simulink model "TST_InjSys_Co"  (R2016b)
settings: Solver=FixedStepDiscrete  StartTime=0.0  StopTime=simTime  FixedStep=sampleTime  RelTol=1e-3
values from neighbouring files (symbols this model uses):
  testCase = 1    [initTST_InjSys_Co_001.m]    (also in initTST_InjSys_Co_002.m = 2; initTST_InjSys_Co_003.m = 3; initTST_InjSys_Co_004.m = 4)
libraries: simulink x33, UnitTest_Lib x28
settings Model: Creator=zhengjinyan  LastModifiedBy=zhengjinyan
settings DebuggingCC: SignalRangeChecking=error

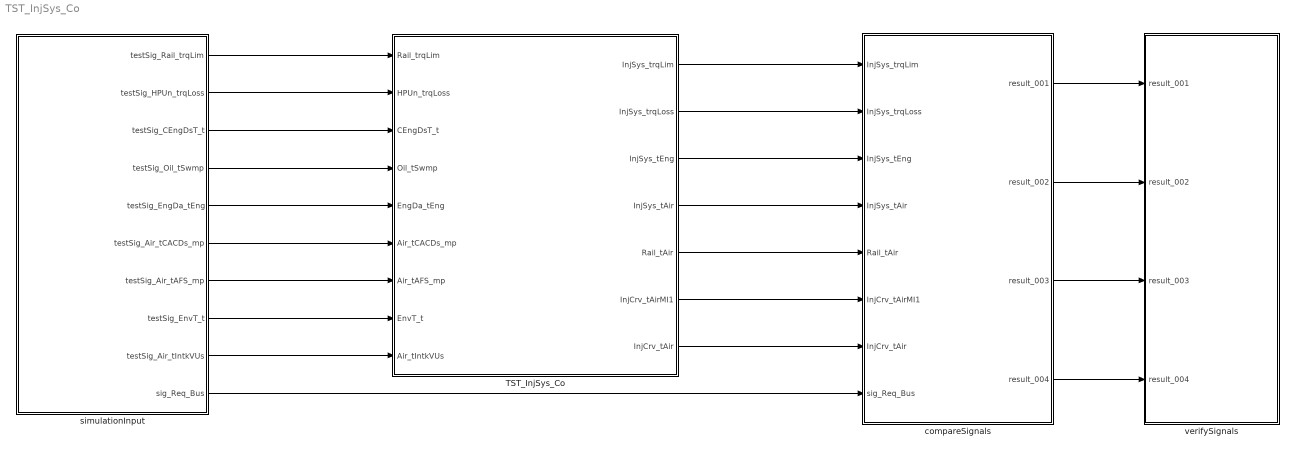
== system TST_InjSys_Co ==
  TST_InjSys_Co : Subsystem
  compareSignals : Subsystem
  simulationInput : Subsystem
  verifySignals : Subsystem
  wires:
  simulationInput/1(testSig_Rail_trqLim) -> TST_InjSys_Co/1(Rail_trqLim)
  simulationInput/2(testSig_HPUn_trqLoss) -> TST_InjSys_Co/2(HPUn_trqLoss)
  simulationInput/3(testSig_CEngDsT_t) -> TST_InjSys_Co/3(CEngDsT_t)
  simulationInput/4(testSig_Oil_tSwmp) -> TST_InjSys_Co/4(Oil_tSwmp)
  simulationInput/5(testSig_EngDa_tEng) -> TST_InjSys_Co/5(EngDa_tEng)
  simulationInput/6(testSig_Air_tCACDs_mp) -> TST_InjSys_Co/6(Air_tCACDs_mp)
  simulationInput/7(testSig_Air_tAFS_mp) -> TST_InjSys_Co/7(Air_tAFS_mp)
  simulationInput/8(testSig_EnvT_t) -> TST_InjSys_Co/8(EnvT_t)
  simulationInput/9(testSig_Air_tIntkVUs) -> TST_InjSys_Co/9(Air_tIntkVUs)
  TST_InjSys_Co/1(InjSys_trqLim) -> compareSignals/1(InjSys_trqLim)
  TST_InjSys_Co/2(InjSys_trqLoss) -> compareSignals/2(InjSys_trqLoss)
  TST_InjSys_Co/3(InjSys_tEng) -> compareSignals/3(InjSys_tEng)
  TST_InjSys_Co/4(InjSys_tAir) -> compareSignals/4(InjSys_tAir)
  TST_InjSys_Co/5(Rail_tAir) -> compareSignals/5(Rail_tAir)
  TST_InjSys_Co/6(InjCrv_tAirMI1) -> compareSignals/6(InjCrv_tAirMI1)
  TST_InjSys_Co/7(InjCrv_tAir) -> compareSignals/7(InjCrv_tAir)
  simulationInput/10(sig_Req_Bus) -> compareSignals/8(sig_Req_Bus)
  compareSignals/1(result_001) -> verifySignals/1(result_001)
  compareSignals/2(result_002) -> verifySignals/2(result_002)
  compareSignals/3(result_003) -> verifySignals/3(result_003)
  compareSignals/4(result_004) -> verifySignals/4(result_004)

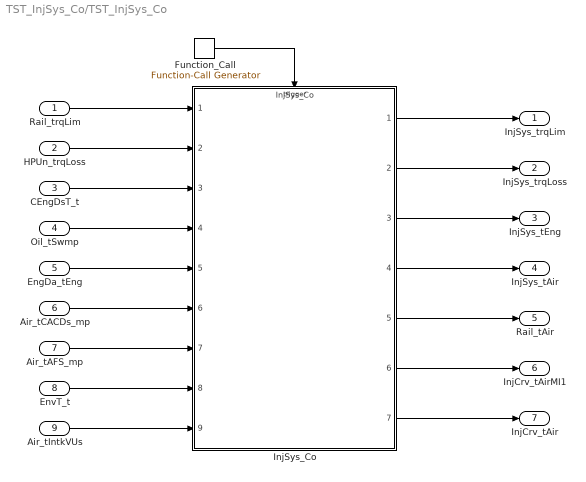
== system TST_InjSys_Co/TST_InjSys_Co ==
  Rail_trqLim : Inport
  HPUn_trqLoss : Inport  Port=2
  CEngDsT_t : Inport  Port=3
  Oil_tSwmp : Inport  Port=4
  EngDa_tEng : Inport  Port=5
  Air_tCACDs_mp : Inport  Port=6
  Air_tAFS_mp : Inport  Port=7
  EnvT_t : Inport  Port=8
  Air_tIntkVUs : Inport  Port=9
  Function_Call : simulink/Ports & Subsystems/Function-Call Generator  sample_time=sampleTime  numberOfIterations=1
  InjSys_Co : ModelReference  ModelNameDialog=InjSys_Co  SimulationMode=Normal  ModelReferenceVersion=1.12  TriggerPortName=function  TriggerPortTriggerType=function-call  TriggerPortStatesWhenEnabling=held
  InjSys_trqLim : Outport
  InjSys_trqLoss : Outport  Port=2
  InjSys_tEng : Outport  Port=3
  InjSys_tAir : Outport  Port=4
  Rail_tAir : Outport  Port=5
  InjCrv_tAirMI1 : Outport  Port=6
  InjCrv_tAir : Outport  Port=7
  wires:
  Function_Call/1 -> InjSys_Co/Trigger
  Rail_trqLim/1 -> InjSys_Co/1
  HPUn_trqLoss/1 -> InjSys_Co/2
  CEngDsT_t/1 -> InjSys_Co/3
  Oil_tSwmp/1 -> InjSys_Co/4
  EngDa_tEng/1 -> InjSys_Co/5
  Air_tCACDs_mp/1 -> InjSys_Co/6
  Air_tAFS_mp/1 -> InjSys_Co/7
  EnvT_t/1 -> InjSys_Co/8
  Air_tIntkVUs/1 -> InjSys_Co/9
  InjSys_Co/1 -> InjSys_trqLim/1
  InjSys_Co/2 -> InjSys_trqLoss/1
  InjSys_Co/3 -> InjSys_tEng/1
  InjSys_Co/4 -> InjSys_tAir/1
  InjSys_Co/5 -> Rail_tAir/1
  InjSys_Co/6 -> InjCrv_tAirMI1/1
  InjSys_Co/7 -> InjCrv_tAir/1

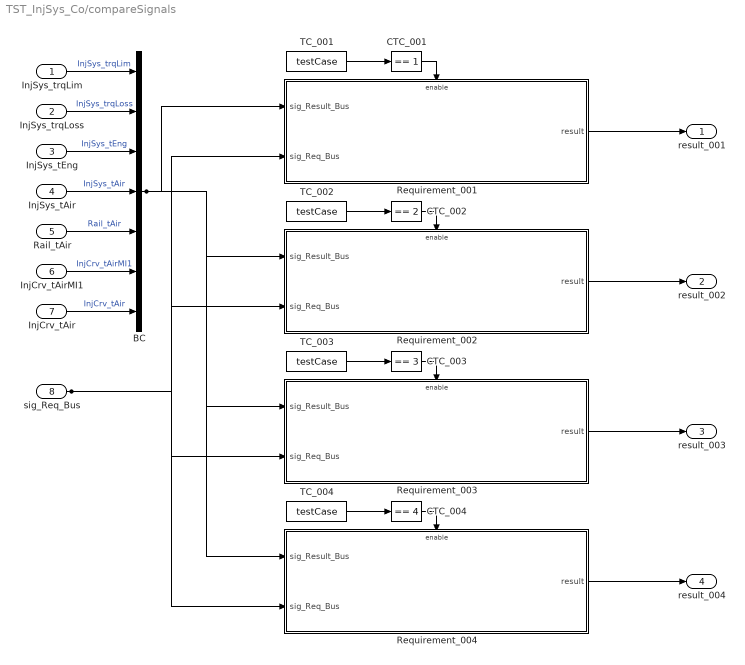
== system TST_InjSys_Co/compareSignals ==
  InjSys_trqLim : Inport
  InjSys_trqLoss : Inport  Port=2
  InjSys_tEng : Inport  Port=3
  InjSys_tAir : Inport  Port=4
  Rail_tAir : Inport  Port=5
  InjCrv_tAirMI1 : Inport  Port=6
  InjCrv_tAir : Inport  Port=7
  sig_Req_Bus : Inport  Port=8
  BC : BusCreator  Inputs=7
  CTC_001 : simulink/Logic and Bit Operations/Compare To Constant  relop===  const=1  OutDataTypeStr=boolean
  CTC_002 : simulink/Logic and Bit Operations/Compare To Constant  relop===  const=2  OutDataTypeStr=boolean
  CTC_003 : simulink/Logic and Bit Operations/Compare To Constant  relop===  const=3  OutDataTypeStr=boolean
  CTC_004 : simulink/Logic and Bit Operations/Compare To Constant  relop===  const=4  OutDataTypeStr=boolean
  Requirement_001 : Subsystem
  Requirement_002 : Subsystem
  Requirement_003 : Subsystem
  Requirement_004 : Subsystem
  TC_001 : Constant  Value=testCase
  TC_002 : Constant  Value=testCase
  TC_003 : Constant  Value=testCase
  TC_004 : Constant  Value=testCase
  result_001 : Outport
  result_002 : Outport  Port=2
  result_003 : Outport  Port=3
  result_004 : Outport  Port=4
  wires:
  InjSys_trqLim/1 -> BC/1  "InjSys_trqLim"
  InjSys_trqLoss/1 -> BC/2  "InjSys_trqLoss"
  InjSys_tEng/1 -> BC/3  "InjSys_tEng"
  InjSys_tAir/1 -> BC/4  "InjSys_tAir"
  Rail_tAir/1 -> BC/5  "Rail_tAir"
  InjCrv_tAirMI1/1 -> BC/6  "InjCrv_tAirMI1"
  InjCrv_tAir/1 -> BC/7  "InjCrv_tAir"
  TC_001/1 -> CTC_001/1
  CTC_001/1 -> Requirement_001/Enable
  sig_Req_Bus/1 -> Requirement_001/2(sig_Req_Bus), Requirement_002/2(sig_Req_Bus), Requirement_003/2(sig_Req_Bus), Requirement_004/2(sig_Req_Bus)
  BC/1 -> Requirement_001/1(sig_Result_Bus), Requirement_002/1(sig_Result_Bus), Requirement_003/1(sig_Result_Bus), Requirement_004/1(sig_Result_Bus)
  Requirement_001/1(result) -> result_001/1
  TC_002/1 -> CTC_002/1
  CTC_002/1 -> Requirement_002/Enable
  Requirement_002/1(result) -> result_002/1
  TC_003/1 -> CTC_003/1
  CTC_003/1 -> Requirement_003/Enable
  Requirement_003/1(result) -> result_003/1
  TC_004/1 -> CTC_004/1
  CTC_004/1 -> Requirement_004/Enable
  Requirement_004/1(result) -> result_004/1

== system TST_InjSys_Co/simulationInput ==
  BS : BusSelector  OutputSignals=testSig_Rail_trqLim,testSig_HPUn_trqLoss,testSig_CEngDsT_t,testSig_Oil_tSwmp,testSig_EngDa_tEng,testSig_Air_tCACDs_mp,testSig_Air_tAFS_mp,testSig_EnvT_t,testSig_Air_tIntkVUs
  MPSw : MultiPortSwitch  Inputs=4  SaturateOnIntegerOverflow=on  InputSameDT=on
  TestCase : Constant  Value=testCase
  testSignals_R001 : Subsystem
  testSignals_R002 : Subsystem
  testSignals_R003 : Subsystem
  testSignals_R004 : Subsystem
  testSig_Rail_trqLim : Outport
  testSig_HPUn_trqLoss : Outport  Port=2
  testSig_CEngDsT_t : Outport  Port=3
  testSig_Oil_tSwmp : Outport  Port=4
  testSig_EngDa_tEng : Outport  Port=5
  testSig_Air_tCACDs_mp : Outport  Port=6
  testSig_Air_tAFS_mp : Outport  Port=7
  testSig_EnvT_t : Outport  Port=8
  testSig_Air_tIntkVUs : Outport  Port=9
  sig_Req_Bus : Outport  Port=10
  wires:
  BS/1 -> testSig_Rail_trqLim/1  "<testSig_Rail_trqLim>"
  BS/2 -> testSig_HPUn_trqLoss/1  "<testSig_HPUn_trqLoss>"
  BS/3 -> testSig_CEngDsT_t/1  "<testSig_CEngDsT_t>"
  BS/4 -> testSig_Oil_tSwmp/1  "<testSig_Oil_tSwmp>"
  BS/5 -> testSig_EngDa_tEng/1  "<testSig_EngDa_tEng>"
  BS/6 -> testSig_Air_tCACDs_mp/1  "<testSig_Air_tCACDs_mp>"
  BS/7 -> testSig_Air_tAFS_mp/1  "<testSig_Air_tAFS_mp>"
  BS/8 -> testSig_EnvT_t/1  "<testSig_EnvT_t>"
  BS/9 -> testSig_Air_tIntkVUs/1  "<testSig_Air_tIntkVUs>"
  MPSw/1 -> BS/1, sig_Req_Bus/1
  TestCase/1 -> MPSw/1
  testSignals_R001/1(testSignals) -> MPSw/2
  testSignals_R002/1(testSignals) -> MPSw/3
  testSignals_R003/1(testSignals) -> MPSw/4
  testSignals_R004/1(testSignals) -> MPSw/5

== system TST_InjSys_Co/verifySignals ==
  result_001 : Inport
  result_002 : Inport  Port=2
  result_003 : Inport  Port=3
  result_004 : Inport  Port=4
  Assertion_001 : Assertion  Enabled=off
  Assertion_002 : Assertion  Enabled=off
  Assertion_003 : Assertion  Enabled=off
  Assertion_004 : Assertion  Enabled=off
  wires:
  result_001/1 -> Assertion_001/1
  result_002/1 -> Assertion_002/1
  result_003/1 -> Assertion_003/1
  result_004/1 -> Assertion_004/1

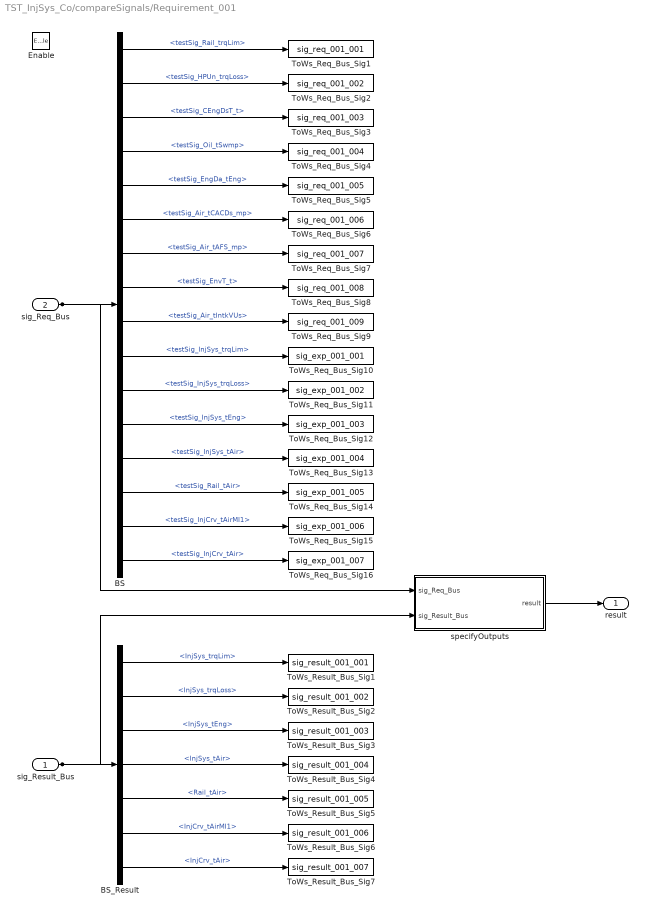
== system TST_InjSys_Co/compareSignals/Requirement_001 ==
  sig_Result_Bus : Inport
  sig_Req_Bus : Inport  Port=2
  Enable : EnablePort
  BS : BusSelector  OutputSignals=testSig_Rail_trqLim,testSig_HPUn_trqLoss,testSig_CEngDsT_t,testSig_Oil_tSwmp,testSig_EngDa_tEng,testSig_Air_tCACDs_mp,testSig_Air_tAFS_mp,testSig_EnvT_t,testSig_Air_tIntkVUs,testSig_InjSys_trqLim,testSig_InjSys_trqLoss,testSig_InjSys_tEng,testSig_InjSys_tAir,testSig_Rail_tAir,testSig_InjCrv_tAirMI1,testSig_InjCrv_tAir
  BS_Result : BusSelector  OutputSignals=InjSys_trqLim,InjSys_trqLoss,InjSys_tEng,InjSys_tAir,Rail_tAir,InjCrv_tAirMI1,InjCrv_tAir
  ToWs_Req_Bus_Sig1 : ToWorkspace  VariableName=sig_req_001_001  SaveFormat=Structure With Time
  ToWs_Req_Bus_Sig10 : ToWorkspace  VariableName=sig_exp_001_001  SaveFormat=Structure With Time
  ToWs_Req_Bus_Sig11 : ToWorkspace  VariableName=sig_exp_001_002  SaveFormat=Structure With Time
  ToWs_Req_Bus_Sig12 : ToWorkspace  VariableName=sig_exp_001_003  SaveFormat=Structure With Time
  ToWs_Req_Bus_Sig13 : ToWorkspace  VariableName=sig_exp_001_004  SaveFormat=Structure With Time
  ToWs_Req_Bus_Sig14 : ToWorkspace  VariableName=sig_exp_001_005  SaveFormat=Structure With Time
  ToWs_Req_Bus_Sig15 : ToWorkspace  VariableName=sig_exp_001_006  SaveFormat=Structure With Time
  ToWs_Req_Bus_Sig16 : ToWorkspace  VariableName=sig_exp_001_007  SaveFormat=Structure With Time
  ToWs_Req_Bus_Sig2 : ToWorkspace  VariableName=sig_req_001_002  SaveFormat=Structure With Time
  ToWs_Req_Bus_Sig3 : ToWorkspace  VariableName=sig_req_001_003  SaveFormat=Structure With Time
  ToWs_Req_Bus_Sig4 : ToWorkspace  VariableName=sig_req_001_004  SaveFormat=Structure With Time
  ToWs_Req_Bus_Sig5 : ToWorkspace  VariableName=sig_req_001_005  SaveFormat=Structure With Time
  ToWs_Req_Bus_Sig6 : ToWorkspace  VariableName=sig_req_001_006  SaveFormat=Structure With Time
  ToWs_Req_Bus_Sig7 : ToWorkspace  VariableName=sig_req_001_007  SaveFormat=Structure With Time
  ToWs_Req_Bus_Sig8 : ToWorkspace  VariableName=sig_req_001_008  SaveFormat=Structure With Time
  ToWs_Req_Bus_Sig9 : ToWorkspace  VariableName=sig_req_001_009  SaveFormat=Structure With Time
  ToWs_Result_Bus_Sig1 : ToWorkspace  VariableName=sig_result_001_001  SaveFormat=Structure With Time
  ToWs_Result_Bus_Sig2 : ToWorkspace  VariableName=sig_result_001_002  SaveFormat=Structure With Time
  ToWs_Result_Bus_Sig3 : ToWorkspace  VariableName=sig_result_001_003  SaveFormat=Structure With Time
  ToWs_Result_Bus_Sig4 : ToWorkspace  VariableName=sig_result_001_004  SaveFormat=Structure With Time
  ToWs_Result_Bus_Sig5 : ToWorkspace  VariableName=sig_result_001_005  SaveFormat=Structure With Time
  ToWs_Result_Bus_Sig6 : ToWorkspace  VariableName=sig_result_001_006  SaveFormat=Structure With Time
  ToWs_Result_Bus_Sig7 : ToWorkspace  VariableName=sig_result_001_007  SaveFormat=Structure With Time
  specifyOutputs : Subsystem
  result : Outport
  wires:
  sig_Req_Bus/1 -> BS/1, specifyOutputs/1(sig_Req_Bus)
  BS/1 -> ToWs_Req_Bus_Sig1/1  "<testSig_Rail_trqLim>"
  BS/2 -> ToWs_Req_Bus_Sig2/1  "<testSig_HPUn_trqLoss>"
  BS/3 -> ToWs_Req_Bus_Sig3/1  "<testSig_CEngDsT_t>"
  BS/4 -> ToWs_Req_Bus_Sig4/1  "<testSig_Oil_tSwmp>"
  BS/5 -> ToWs_Req_Bus_Sig5/1  "<testSig_EngDa_tEng>"
  BS/6 -> ToWs_Req_Bus_Sig6/1  "<testSig_Air_tCACDs_mp>"
  BS/7 -> ToWs_Req_Bus_Sig7/1  "<testSig_Air_tAFS_mp>"
  BS/8 -> ToWs_Req_Bus_Sig8/1  "<testSig_EnvT_t>"
  BS/9 -> ToWs_Req_Bus_Sig9/1  "<testSig_Air_tIntkVUs>"
  BS/10 -> ToWs_Req_Bus_Sig10/1  "<testSig_InjSys_trqLim>"
  BS/11 -> ToWs_Req_Bus_Sig11/1  "<testSig_InjSys_trqLoss>"
  BS/12 -> ToWs_Req_Bus_Sig12/1  "<testSig_InjSys_tEng>"
  BS/13 -> ToWs_Req_Bus_Sig13/1  "<testSig_InjSys_tAir>"
  BS/14 -> ToWs_Req_Bus_Sig14/1  "<testSig_Rail_tAir>"
  BS/15 -> ToWs_Req_Bus_Sig15/1  "<testSig_InjCrv_tAirMI1>"
  BS/16 -> ToWs_Req_Bus_Sig16/1  "<testSig_InjCrv_tAir>"
  sig_Result_Bus/1 -> BS_Result/1, specifyOutputs/2(sig_Result_Bus)
  BS_Result/1 -> ToWs_Result_Bus_Sig1/1  "<InjSys_trqLim>"
  BS_Result/2 -> ToWs_Result_Bus_Sig2/1  "<InjSys_trqLoss>"
  BS_Result/3 -> ToWs_Result_Bus_Sig3/1  "<InjSys_tEng>"
  BS_Result/4 -> ToWs_Result_Bus_Sig4/1  "<InjSys_tAir>"
  BS_Result/5 -> ToWs_Result_Bus_Sig5/1  "<Rail_tAir>"
  BS_Result/6 -> ToWs_Result_Bus_Sig6/1  "<InjCrv_tAirMI1>"
  BS_Result/7 -> ToWs_Result_Bus_Sig7/1  "<InjCrv_tAir>"
  specifyOutputs/1(result) -> result/1

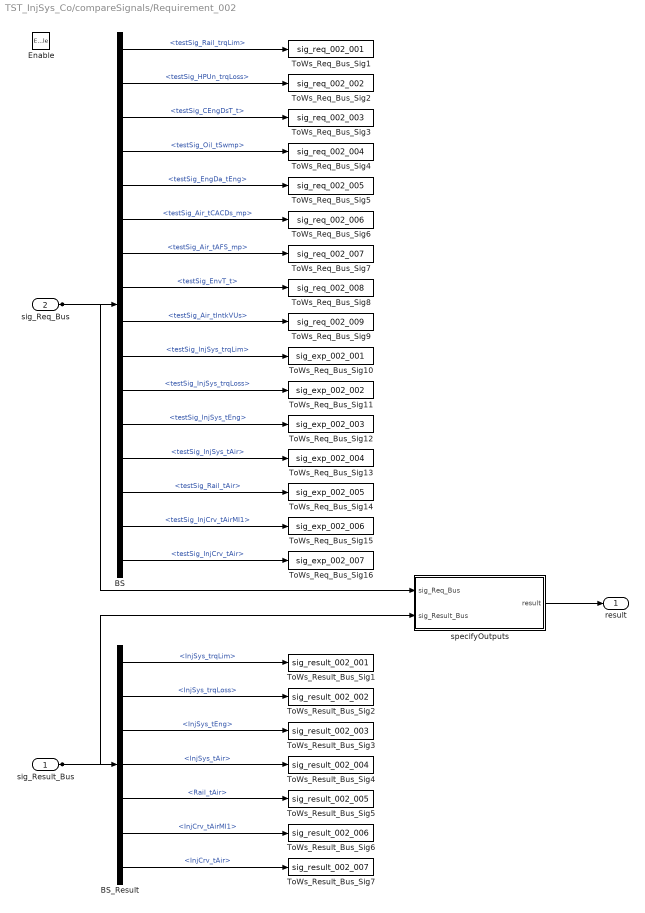
== system TST_InjSys_Co/compareSignals/Requirement_002 ==
  sig_Result_Bus : Inport
  sig_Req_Bus : Inport  Port=2
  Enable : EnablePort
  BS : BusSelector  OutputSignals=testSig_Rail_trqLim,testSig_HPUn_trqLoss,testSig_CEngDsT_t,testSig_Oil_tSwmp,testSig_EngDa_tEng,testSig_Air_tCACDs_mp,testSig_Air_tAFS_mp,testSig_EnvT_t,testSig_Air_tIntkVUs,testSig_InjSys_trqLim,testSig_InjSys_trqLoss,testSig_InjSys_tEng,testSig_InjSys_tAir,testSig_Rail_tAir,testSig_InjCrv_tAirMI1,testSig_InjCrv_tAir
  BS_Result : BusSelector  OutputSignals=InjSys_trqLim,InjSys_trqLoss,InjSys_tEng,InjSys_tAir,Rail_tAir,InjCrv_tAirMI1,InjCrv_tAir
  ToWs_Req_Bus_Sig1 : ToWorkspace  VariableName=sig_req_002_001  SaveFormat=Structure With Time
  ToWs_Req_Bus_Sig10 : ToWorkspace  VariableName=sig_exp_002_001  SaveFormat=Structure With Time
  ToWs_Req_Bus_Sig11 : ToWorkspace  VariableName=sig_exp_002_002  SaveFormat=Structure With Time
  ToWs_Req_Bus_Sig12 : ToWorkspace  VariableName=sig_exp_002_003  SaveFormat=Structure With Time
  ToWs_Req_Bus_Sig13 : ToWorkspace  VariableName=sig_exp_002_004  SaveFormat=Structure With Time
  ToWs_Req_Bus_Sig14 : ToWorkspace  VariableName=sig_exp_002_005  SaveFormat=Structure With Time
  ToWs_Req_Bus_Sig15 : ToWorkspace  VariableName=sig_exp_002_006  SaveFormat=Structure With Time
  ToWs_Req_Bus_Sig16 : ToWorkspace  VariableName=sig_exp_002_007  SaveFormat=Structure With Time
  ToWs_Req_Bus_Sig2 : ToWorkspace  VariableName=sig_req_002_002  SaveFormat=Structure With Time
  ToWs_Req_Bus_Sig3 : ToWorkspace  VariableName=sig_req_002_003  SaveFormat=Structure With Time
  ToWs_Req_Bus_Sig4 : ToWorkspace  VariableName=sig_req_002_004  SaveFormat=Structure With Time
  ToWs_Req_Bus_Sig5 : ToWorkspace  VariableName=sig_req_002_005  SaveFormat=Structure With Time
  ToWs_Req_Bus_Sig6 : ToWorkspace  VariableName=sig_req_002_006  SaveFormat=Structure With Time
  ToWs_Req_Bus_Sig7 : ToWorkspace  VariableName=sig_req_002_007  SaveFormat=Structure With Time
  ToWs_Req_Bus_Sig8 : ToWorkspace  VariableName=sig_req_002_008  SaveFormat=Structure With Time
  ToWs_Req_Bus_Sig9 : ToWorkspace  VariableName=sig_req_002_009  SaveFormat=Structure With Time
  ToWs_Result_Bus_Sig1 : ToWorkspace  VariableName=sig_result_002_001  SaveFormat=Structure With Time
  ToWs_Result_Bus_Sig2 : ToWorkspace  VariableName=sig_result_002_002  SaveFormat=Structure With Time
  ToWs_Result_Bus_Sig3 : ToWorkspace  VariableName=sig_result_002_003  SaveFormat=Structure With Time
  ToWs_Result_Bus_Sig4 : ToWorkspace  VariableName=sig_result_002_004  SaveFormat=Structure With Time
  ToWs_Result_Bus_Sig5 : ToWorkspace  VariableName=sig_result_002_005  SaveFormat=Structure With Time
  ToWs_Result_Bus_Sig6 : ToWorkspace  VariableName=sig_result_002_006  SaveFormat=Structure With Time
  ToWs_Result_Bus_Sig7 : ToWorkspace  VariableName=sig_result_002_007  SaveFormat=Structure With Time
  specifyOutputs : Subsystem
  result : Outport
  wires:
  sig_Req_Bus/1 -> BS/1, specifyOutputs/1(sig_Req_Bus)
  BS/1 -> ToWs_Req_Bus_Sig1/1  "<testSig_Rail_trqLim>"
  BS/2 -> ToWs_Req_Bus_Sig2/1  "<testSig_HPUn_trqLoss>"
  BS/3 -> ToWs_Req_Bus_Sig3/1  "<testSig_CEngDsT_t>"
  BS/4 -> ToWs_Req_Bus_Sig4/1  "<testSig_Oil_tSwmp>"
  BS/5 -> ToWs_Req_Bus_Sig5/1  "<testSig_EngDa_tEng>"
  BS/6 -> ToWs_Req_Bus_Sig6/1  "<testSig_Air_tCACDs_mp>"
  BS/7 -> ToWs_Req_Bus_Sig7/1  "<testSig_Air_tAFS_mp>"
  BS/8 -> ToWs_Req_Bus_Sig8/1  "<testSig_EnvT_t>"
  BS/9 -> ToWs_Req_Bus_Sig9/1  "<testSig_Air_tIntkVUs>"
  BS/10 -> ToWs_Req_Bus_Sig10/1  "<testSig_InjSys_trqLim>"
  BS/11 -> ToWs_Req_Bus_Sig11/1  "<testSig_InjSys_trqLoss>"
  BS/12 -> ToWs_Req_Bus_Sig12/1  "<testSig_InjSys_tEng>"
  BS/13 -> ToWs_Req_Bus_Sig13/1  "<testSig_InjSys_tAir>"
  BS/14 -> ToWs_Req_Bus_Sig14/1  "<testSig_Rail_tAir>"
  BS/15 -> ToWs_Req_Bus_Sig15/1  "<testSig_InjCrv_tAirMI1>"
  BS/16 -> ToWs_Req_Bus_Sig16/1  "<testSig_InjCrv_tAir>"
  sig_Result_Bus/1 -> BS_Result/1, specifyOutputs/2(sig_Result_Bus)
  BS_Result/1 -> ToWs_Result_Bus_Sig1/1  "<InjSys_trqLim>"
  BS_Result/2 -> ToWs_Result_Bus_Sig2/1  "<InjSys_trqLoss>"
  BS_Result/3 -> ToWs_Result_Bus_Sig3/1  "<InjSys_tEng>"
  BS_Result/4 -> ToWs_Result_Bus_Sig4/1  "<InjSys_tAir>"
  BS_Result/5 -> ToWs_Result_Bus_Sig5/1  "<Rail_tAir>"
  BS_Result/6 -> ToWs_Result_Bus_Sig6/1  "<InjCrv_tAirMI1>"
  BS_Result/7 -> ToWs_Result_Bus_Sig7/1  "<InjCrv_tAir>"
  specifyOutputs/1(result) -> result/1

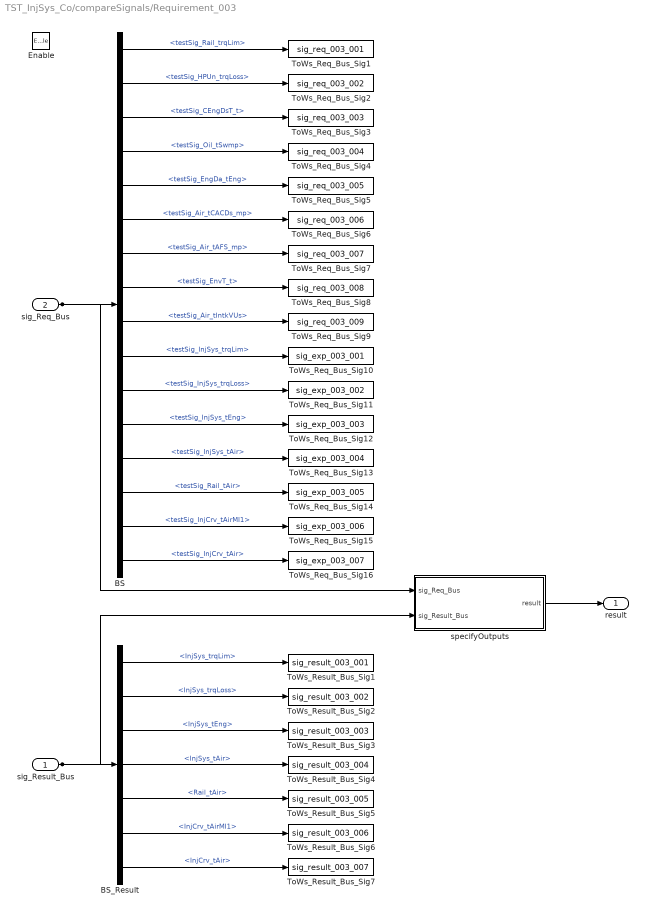
== system TST_InjSys_Co/compareSignals/Requirement_003 ==
  sig_Result_Bus : Inport
  sig_Req_Bus : Inport  Port=2
  Enable : EnablePort
  BS : BusSelector  OutputSignals=testSig_Rail_trqLim,testSig_HPUn_trqLoss,testSig_CEngDsT_t,testSig_Oil_tSwmp,testSig_EngDa_tEng,testSig_Air_tCACDs_mp,testSig_Air_tAFS_mp,testSig_EnvT_t,testSig_Air_tIntkVUs,testSig_InjSys_trqLim,testSig_InjSys_trqLoss,testSig_InjSys_tEng,testSig_InjSys_tAir,testSig_Rail_tAir,testSig_InjCrv_tAirMI1,testSig_InjCrv_tAir
  BS_Result : BusSelector  OutputSignals=InjSys_trqLim,InjSys_trqLoss,InjSys_tEng,InjSys_tAir,Rail_tAir,InjCrv_tAirMI1,InjCrv_tAir
  ToWs_Req_Bus_Sig1 : ToWorkspace  VariableName=sig_req_003_001  SaveFormat=Structure With Time
  ToWs_Req_Bus_Sig10 : ToWorkspace  VariableName=sig_exp_003_001  SaveFormat=Structure With Time
  ToWs_Req_Bus_Sig11 : ToWorkspace  VariableName=sig_exp_003_002  SaveFormat=Structure With Time
  ToWs_Req_Bus_Sig12 : ToWorkspace  VariableName=sig_exp_003_003  SaveFormat=Structure With Time
  ToWs_Req_Bus_Sig13 : ToWorkspace  VariableName=sig_exp_003_004  SaveFormat=Structure With Time
  ToWs_Req_Bus_Sig14 : ToWorkspace  VariableName=sig_exp_003_005  SaveFormat=Structure With Time
  ToWs_Req_Bus_Sig15 : ToWorkspace  VariableName=sig_exp_003_006  SaveFormat=Structure With Time
  ToWs_Req_Bus_Sig16 : ToWorkspace  VariableName=sig_exp_003_007  SaveFormat=Structure With Time
  ToWs_Req_Bus_Sig2 : ToWorkspace  VariableName=sig_req_003_002  SaveFormat=Structure With Time
  ToWs_Req_Bus_Sig3 : ToWorkspace  VariableName=sig_req_003_003  SaveFormat=Structure With Time
  ToWs_Req_Bus_Sig4 : ToWorkspace  VariableName=sig_req_003_004  SaveFormat=Structure With Time
  ToWs_Req_Bus_Sig5 : ToWorkspace  VariableName=sig_req_003_005  SaveFormat=Structure With Time
  ToWs_Req_Bus_Sig6 : ToWorkspace  VariableName=sig_req_003_006  SaveFormat=Structure With Time
  ToWs_Req_Bus_Sig7 : ToWorkspace  VariableName=sig_req_003_007  SaveFormat=Structure With Time
  ToWs_Req_Bus_Sig8 : ToWorkspace  VariableName=sig_req_003_008  SaveFormat=Structure With Time
  ToWs_Req_Bus_Sig9 : ToWorkspace  VariableName=sig_req_003_009  SaveFormat=Structure With Time
  ToWs_Result_Bus_Sig1 : ToWorkspace  VariableName=sig_result_003_001  SaveFormat=Structure With Time
  ToWs_Result_Bus_Sig2 : ToWorkspace  VariableName=sig_result_003_002  SaveFormat=Structure With Time
  ToWs_Result_Bus_Sig3 : ToWorkspace  VariableName=sig_result_003_003  SaveFormat=Structure With Time
  ToWs_Result_Bus_Sig4 : ToWorkspace  VariableName=sig_result_003_004  SaveFormat=Structure With Time
  ToWs_Result_Bus_Sig5 : ToWorkspace  VariableName=sig_result_003_005  SaveFormat=Structure With Time
  ToWs_Result_Bus_Sig6 : ToWorkspace  VariableName=sig_result_003_006  SaveFormat=Structure With Time
  ToWs_Result_Bus_Sig7 : ToWorkspace  VariableName=sig_result_003_007  SaveFormat=Structure With Time
  specifyOutputs : Subsystem
  result : Outport
  wires:
  sig_Req_Bus/1 -> BS/1, specifyOutputs/1(sig_Req_Bus)
  BS/1 -> ToWs_Req_Bus_Sig1/1  "<testSig_Rail_trqLim>"
  BS/2 -> ToWs_Req_Bus_Sig2/1  "<testSig_HPUn_trqLoss>"
  BS/3 -> ToWs_Req_Bus_Sig3/1  "<testSig_CEngDsT_t>"
  BS/4 -> ToWs_Req_Bus_Sig4/1  "<testSig_Oil_tSwmp>"
  BS/5 -> ToWs_Req_Bus_Sig5/1  "<testSig_EngDa_tEng>"
  BS/6 -> ToWs_Req_Bus_Sig6/1  "<testSig_Air_tCACDs_mp>"
  BS/7 -> ToWs_Req_Bus_Sig7/1  "<testSig_Air_tAFS_mp>"
  BS/8 -> ToWs_Req_Bus_Sig8/1  "<testSig_EnvT_t>"
  BS/9 -> ToWs_Req_Bus_Sig9/1  "<testSig_Air_tIntkVUs>"
  BS/10 -> ToWs_Req_Bus_Sig10/1  "<testSig_InjSys_trqLim>"
  BS/11 -> ToWs_Req_Bus_Sig11/1  "<testSig_InjSys_trqLoss>"
  BS/12 -> ToWs_Req_Bus_Sig12/1  "<testSig_InjSys_tEng>"
  BS/13 -> ToWs_Req_Bus_Sig13/1  "<testSig_InjSys_tAir>"
  BS/14 -> ToWs_Req_Bus_Sig14/1  "<testSig_Rail_tAir>"
  BS/15 -> ToWs_Req_Bus_Sig15/1  "<testSig_InjCrv_tAirMI1>"
  BS/16 -> ToWs_Req_Bus_Sig16/1  "<testSig_InjCrv_tAir>"
  sig_Result_Bus/1 -> BS_Result/1, specifyOutputs/2(sig_Result_Bus)
  BS_Result/1 -> ToWs_Result_Bus_Sig1/1  "<InjSys_trqLim>"
  BS_Result/2 -> ToWs_Result_Bus_Sig2/1  "<InjSys_trqLoss>"
  BS_Result/3 -> ToWs_Result_Bus_Sig3/1  "<InjSys_tEng>"
  BS_Result/4 -> ToWs_Result_Bus_Sig4/1  "<InjSys_tAir>"
  BS_Result/5 -> ToWs_Result_Bus_Sig5/1  "<Rail_tAir>"
  BS_Result/6 -> ToWs_Result_Bus_Sig6/1  "<InjCrv_tAirMI1>"
  BS_Result/7 -> ToWs_Result_Bus_Sig7/1  "<InjCrv_tAir>"
  specifyOutputs/1(result) -> result/1

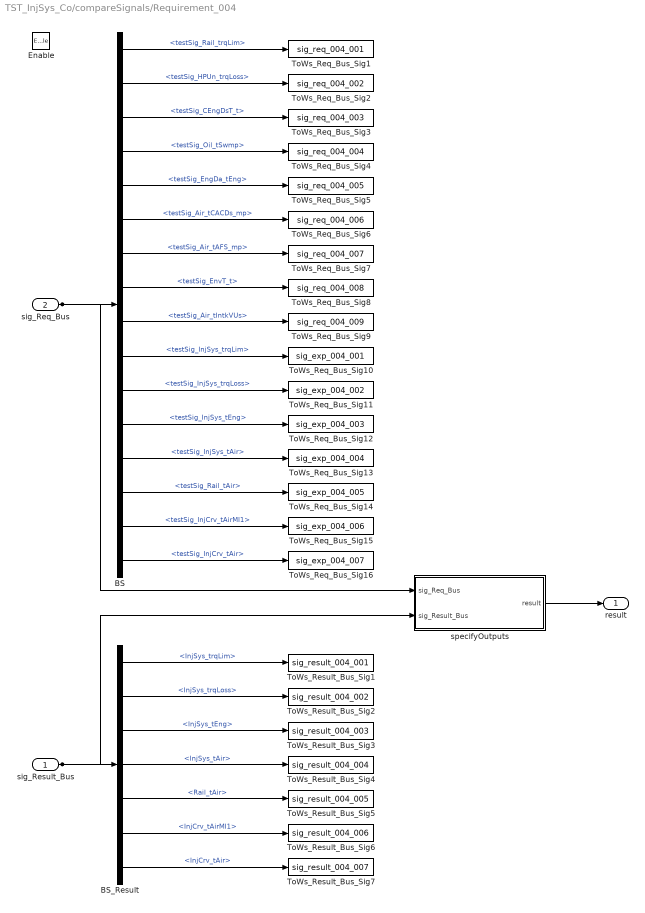
== system TST_InjSys_Co/compareSignals/Requirement_004 ==
  sig_Result_Bus : Inport
  sig_Req_Bus : Inport  Port=2
  Enable : EnablePort
  BS : BusSelector  OutputSignals=testSig_Rail_trqLim,testSig_HPUn_trqLoss,testSig_CEngDsT_t,testSig_Oil_tSwmp,testSig_EngDa_tEng,testSig_Air_tCACDs_mp,testSig_Air_tAFS_mp,testSig_EnvT_t,testSig_Air_tIntkVUs,testSig_InjSys_trqLim,testSig_InjSys_trqLoss,testSig_InjSys_tEng,testSig_InjSys_tAir,testSig_Rail_tAir,testSig_InjCrv_tAirMI1,testSig_InjCrv_tAir
  BS_Result : BusSelector  OutputSignals=InjSys_trqLim,InjSys_trqLoss,InjSys_tEng,InjSys_tAir,Rail_tAir,InjCrv_tAirMI1,InjCrv_tAir
  ToWs_Req_Bus_Sig1 : ToWorkspace  VariableName=sig_req_004_001  SaveFormat=Structure With Time
  ToWs_Req_Bus_Sig10 : ToWorkspace  VariableName=sig_exp_004_001  SaveFormat=Structure With Time
  ToWs_Req_Bus_Sig11 : ToWorkspace  VariableName=sig_exp_004_002  SaveFormat=Structure With Time
  ToWs_Req_Bus_Sig12 : ToWorkspace  VariableName=sig_exp_004_003  SaveFormat=Structure With Time
  ToWs_Req_Bus_Sig13 : ToWorkspace  VariableName=sig_exp_004_004  SaveFormat=Structure With Time
  ToWs_Req_Bus_Sig14 : ToWorkspace  VariableName=sig_exp_004_005  SaveFormat=Structure With Time
  ToWs_Req_Bus_Sig15 : ToWorkspace  VariableName=sig_exp_004_006  SaveFormat=Structure With Time
  ToWs_Req_Bus_Sig16 : ToWorkspace  VariableName=sig_exp_004_007  SaveFormat=Structure With Time
  ToWs_Req_Bus_Sig2 : ToWorkspace  VariableName=sig_req_004_002  SaveFormat=Structure With Time
  ToWs_Req_Bus_Sig3 : ToWorkspace  VariableName=sig_req_004_003  SaveFormat=Structure With Time
  ToWs_Req_Bus_Sig4 : ToWorkspace  VariableName=sig_req_004_004  SaveFormat=Structure With Time
  ToWs_Req_Bus_Sig5 : ToWorkspace  VariableName=sig_req_004_005  SaveFormat=Structure With Time
  ToWs_Req_Bus_Sig6 : ToWorkspace  VariableName=sig_req_004_006  SaveFormat=Structure With Time
  ToWs_Req_Bus_Sig7 : ToWorkspace  VariableName=sig_req_004_007  SaveFormat=Structure With Time
  ToWs_Req_Bus_Sig8 : ToWorkspace  VariableName=sig_req_004_008  SaveFormat=Structure With Time
  ToWs_Req_Bus_Sig9 : ToWorkspace  VariableName=sig_req_004_009  SaveFormat=Structure With Time
  ToWs_Result_Bus_Sig1 : ToWorkspace  VariableName=sig_result_004_001  SaveFormat=Structure With Time
  ToWs_Result_Bus_Sig2 : ToWorkspace  VariableName=sig_result_004_002  SaveFormat=Structure With Time
  ToWs_Result_Bus_Sig3 : ToWorkspace  VariableName=sig_result_004_003  SaveFormat=Structure With Time
  ToWs_Result_Bus_Sig4 : ToWorkspace  VariableName=sig_result_004_004  SaveFormat=Structure With Time
  ToWs_Result_Bus_Sig5 : ToWorkspace  VariableName=sig_result_004_005  SaveFormat=Structure With Time
  ToWs_Result_Bus_Sig6 : ToWorkspace  VariableName=sig_result_004_006  SaveFormat=Structure With Time
  ToWs_Result_Bus_Sig7 : ToWorkspace  VariableName=sig_result_004_007  SaveFormat=Structure With Time
  specifyOutputs : Subsystem
  result : Outport
  wires:
  sig_Req_Bus/1 -> BS/1, specifyOutputs/1(sig_Req_Bus)
  BS/1 -> ToWs_Req_Bus_Sig1/1  "<testSig_Rail_trqLim>"
  BS/2 -> ToWs_Req_Bus_Sig2/1  "<testSig_HPUn_trqLoss>"
  BS/3 -> ToWs_Req_Bus_Sig3/1  "<testSig_CEngDsT_t>"
  BS/4 -> ToWs_Req_Bus_Sig4/1  "<testSig_Oil_tSwmp>"
  BS/5 -> ToWs_Req_Bus_Sig5/1  "<testSig_EngDa_tEng>"
  BS/6 -> ToWs_Req_Bus_Sig6/1  "<testSig_Air_tCACDs_mp>"
  BS/7 -> ToWs_Req_Bus_Sig7/1  "<testSig_Air_tAFS_mp>"
  BS/8 -> ToWs_Req_Bus_Sig8/1  "<testSig_EnvT_t>"
  BS/9 -> ToWs_Req_Bus_Sig9/1  "<testSig_Air_tIntkVUs>"
  BS/10 -> ToWs_Req_Bus_Sig10/1  "<testSig_InjSys_trqLim>"
  BS/11 -> ToWs_Req_Bus_Sig11/1  "<testSig_InjSys_trqLoss>"
  BS/12 -> ToWs_Req_Bus_Sig12/1  "<testSig_InjSys_tEng>"
  BS/13 -> ToWs_Req_Bus_Sig13/1  "<testSig_InjSys_tAir>"
  BS/14 -> ToWs_Req_Bus_Sig14/1  "<testSig_Rail_tAir>"
  BS/15 -> ToWs_Req_Bus_Sig15/1  "<testSig_InjCrv_tAirMI1>"
  BS/16 -> ToWs_Req_Bus_Sig16/1  "<testSig_InjCrv_tAir>"
  sig_Result_Bus/1 -> BS_Result/1, specifyOutputs/2(sig_Result_Bus)
  BS_Result/1 -> ToWs_Result_Bus_Sig1/1  "<InjSys_trqLim>"
  BS_Result/2 -> ToWs_Result_Bus_Sig2/1  "<InjSys_trqLoss>"
  BS_Result/3 -> ToWs_Result_Bus_Sig3/1  "<InjSys_tEng>"
  BS_Result/4 -> ToWs_Result_Bus_Sig4/1  "<InjSys_tAir>"
  BS_Result/5 -> ToWs_Result_Bus_Sig5/1  "<Rail_tAir>"
  BS_Result/6 -> ToWs_Result_Bus_Sig6/1  "<InjCrv_tAirMI1>"
  BS_Result/7 -> ToWs_Result_Bus_Sig7/1  "<InjCrv_tAir>"
  specifyOutputs/1(result) -> result/1

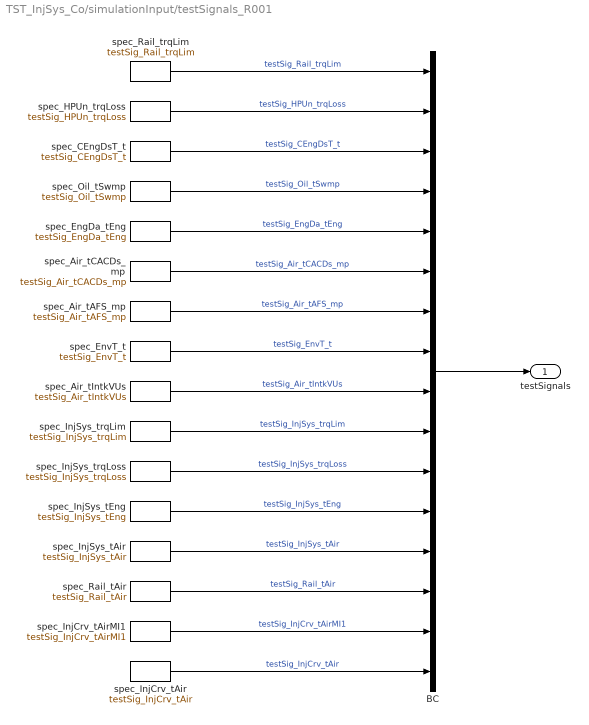
== system TST_InjSys_Co/simulationInput/testSignals_R001 ==
  BC : BusCreator  Inputs=16
  spec_Air_tAFS_mp : FromWorkspace  VariableName=testSig_Air_tAFS_mp  Interpolate=off  OutputAfterFinalValue=Holding final value
  spec_Air_tCACDs_mp : FromWorkspace  VariableName=testSig_Air_tCACDs_mp  Interpolate=off  OutputAfterFinalValue=Holding final value
  spec_Air_tIntkVUs : FromWorkspace  VariableName=testSig_Air_tIntkVUs  Interpolate=off  OutputAfterFinalValue=Holding final value
  spec_CEngDsT_t : FromWorkspace  VariableName=testSig_CEngDsT_t  Interpolate=off  OutputAfterFinalValue=Holding final value
  spec_EngDa_tEng : FromWorkspace  VariableName=testSig_EngDa_tEng  Interpolate=off  OutputAfterFinalValue=Holding final value
  spec_EnvT_t : FromWorkspace  VariableName=testSig_EnvT_t  Interpolate=off  OutputAfterFinalValue=Holding final value
  spec_HPUn_trqLoss : FromWorkspace  VariableName=testSig_HPUn_trqLoss  Interpolate=off  OutputAfterFinalValue=Holding final value
  spec_InjCrv_tAir : FromWorkspace  VariableName=testSig_InjCrv_tAir  Interpolate=off  OutputAfterFinalValue=Holding final value
  spec_InjCrv_tAirMI1 : FromWorkspace  VariableName=testSig_InjCrv_tAirMI1  Interpolate=off  OutputAfterFinalValue=Holding final value
  spec_InjSys_tAir : FromWorkspace  VariableName=testSig_InjSys_tAir  Interpolate=off  OutputAfterFinalValue=Holding final value
  spec_InjSys_tEng : FromWorkspace  VariableName=testSig_InjSys_tEng  Interpolate=off  OutputAfterFinalValue=Holding final value
  spec_InjSys_trqLim : FromWorkspace  VariableName=testSig_InjSys_trqLim  Interpolate=off  OutputAfterFinalValue=Holding final value
  spec_InjSys_trqLoss : FromWorkspace  VariableName=testSig_InjSys_trqLoss  Interpolate=off  OutputAfterFinalValue=Holding final value
  spec_Oil_tSwmp : FromWorkspace  VariableName=testSig_Oil_tSwmp  Interpolate=off  OutputAfterFinalValue=Holding final value
  spec_Rail_tAir : FromWorkspace  VariableName=testSig_Rail_tAir  Interpolate=off  OutputAfterFinalValue=Holding final value
  spec_Rail_trqLim : FromWorkspace  VariableName=testSig_Rail_trqLim  Interpolate=off  OutputAfterFinalValue=Holding final value
  testSignals : Outport
  wires:
  BC/1 -> testSignals/1
  spec_Rail_trqLim/1 -> BC/1  "testSig_Rail_trqLim"
  spec_HPUn_trqLoss/1 -> BC/2  "testSig_HPUn_trqLoss"
  spec_CEngDsT_t/1 -> BC/3  "testSig_CEngDsT_t"
  spec_Oil_tSwmp/1 -> BC/4  "testSig_Oil_tSwmp"
  spec_EngDa_tEng/1 -> BC/5  "testSig_EngDa_tEng"
  spec_Air_tCACDs_mp/1 -> BC/6  "testSig_Air_tCACDs_mp"
  spec_Air_tAFS_mp/1 -> BC/7  "testSig_Air_tAFS_mp"
  spec_EnvT_t/1 -> BC/8  "testSig_EnvT_t"
  spec_Air_tIntkVUs/1 -> BC/9  "testSig_Air_tIntkVUs"
  spec_InjSys_trqLim/1 -> BC/10  "testSig_InjSys_trqLim"
  spec_InjSys_trqLoss/1 -> BC/11  "testSig_InjSys_trqLoss"
  spec_InjSys_tEng/1 -> BC/12  "testSig_InjSys_tEng"
  spec_InjSys_tAir/1 -> BC/13  "testSig_InjSys_tAir"
  spec_Rail_tAir/1 -> BC/14  "testSig_Rail_tAir"
  spec_InjCrv_tAirMI1/1 -> BC/15  "testSig_InjCrv_tAirMI1"
  spec_InjCrv_tAir/1 -> BC/16  "testSig_InjCrv_tAir"

== system TST_InjSys_Co/simulationInput/testSignals_R002 ==
  BC : BusCreator  Inputs=16
  spec_Air_tAFS_mp : FromWorkspace  VariableName=testSig_Air_tAFS_mp  Interpolate=off  OutputAfterFinalValue=Holding final value
  spec_Air_tCACDs_mp : FromWorkspace  VariableName=testSig_Air_tCACDs_mp  Interpolate=off  OutputAfterFinalValue=Holding final value
  spec_Air_tIntkVUs : FromWorkspace  VariableName=testSig_Air_tIntkVUs  Interpolate=off  OutputAfterFinalValue=Holding final value
  spec_CEngDsT_t : FromWorkspace  VariableName=testSig_CEngDsT_t  Interpolate=off  OutputAfterFinalValue=Holding final value
  spec_EngDa_tEng : FromWorkspace  VariableName=testSig_EngDa_tEng  Interpolate=off  OutputAfterFinalValue=Holding final value
  spec_EnvT_t : FromWorkspace  VariableName=testSig_EnvT_t  Interpolate=off  OutputAfterFinalValue=Holding final value
  spec_HPUn_trqLoss : FromWorkspace  VariableName=testSig_HPUn_trqLoss  Interpolate=off  OutputAfterFinalValue=Holding final value
  spec_InjCrv_tAir : FromWorkspace  VariableName=testSig_InjCrv_tAir  Interpolate=off  OutputAfterFinalValue=Holding final value
  spec_InjCrv_tAirMI1 : FromWorkspace  VariableName=testSig_InjCrv_tAirMI1  Interpolate=off  OutputAfterFinalValue=Holding final value
  spec_InjSys_tAir : FromWorkspace  VariableName=testSig_InjSys_tAir  Interpolate=off  OutputAfterFinalValue=Holding final value
  spec_InjSys_tEng : FromWorkspace  VariableName=testSig_InjSys_tEng  Interpolate=off  OutputAfterFinalValue=Holding final value
  spec_InjSys_trqLim : FromWorkspace  VariableName=testSig_InjSys_trqLim  Interpolate=off  OutputAfterFinalValue=Holding final value
  spec_InjSys_trqLoss : FromWorkspace  VariableName=testSig_InjSys_trqLoss  Interpolate=off  OutputAfterFinalValue=Holding final value
  spec_Oil_tSwmp : FromWorkspace  VariableName=testSig_Oil_tSwmp  Interpolate=off  OutputAfterFinalValue=Holding final value
  spec_Rail_tAir : FromWorkspace  VariableName=testSig_Rail_tAir  Interpolate=off  OutputAfterFinalValue=Holding final value
  spec_Rail_trqLim : FromWorkspace  VariableName=testSig_Rail_trqLim  Interpolate=off  OutputAfterFinalValue=Holding final value
  testSignals : Outport
  wires:
  BC/1 -> testSignals/1
  spec_Rail_trqLim/1 -> BC/1  "testSig_Rail_trqLim"
  spec_HPUn_trqLoss/1 -> BC/2  "testSig_HPUn_trqLoss"
  spec_CEngDsT_t/1 -> BC/3  "testSig_CEngDsT_t"
  spec_Oil_tSwmp/1 -> BC/4  "testSig_Oil_tSwmp"
  spec_EngDa_tEng/1 -> BC/5  "testSig_EngDa_tEng"
  spec_Air_tCACDs_mp/1 -> BC/6  "testSig_Air_tCACDs_mp"
  spec_Air_tAFS_mp/1 -> BC/7  "testSig_Air_tAFS_mp"
  spec_EnvT_t/1 -> BC/8  "testSig_EnvT_t"
  spec_Air_tIntkVUs/1 -> BC/9  "testSig_Air_tIntkVUs"
  spec_InjSys_trqLim/1 -> BC/10  "testSig_InjSys_trqLim"
  spec_InjSys_trqLoss/1 -> BC/11  "testSig_InjSys_trqLoss"
  spec_InjSys_tEng/1 -> BC/12  "testSig_InjSys_tEng"
  spec_InjSys_tAir/1 -> BC/13  "testSig_InjSys_tAir"
  spec_Rail_tAir/1 -> BC/14  "testSig_Rail_tAir"
  spec_InjCrv_tAirMI1/1 -> BC/15  "testSig_InjCrv_tAirMI1"
  spec_InjCrv_tAir/1 -> BC/16  "testSig_InjCrv_tAir"

== system TST_InjSys_Co/simulationInput/testSignals_R003 ==
  BC : BusCreator  Inputs=16
  spec_Air_tAFS_mp : FromWorkspace  VariableName=testSig_Air_tAFS_mp  Interpolate=off  OutputAfterFinalValue=Holding final value
  spec_Air_tCACDs_mp : FromWorkspace  VariableName=testSig_Air_tCACDs_mp  Interpolate=off  OutputAfterFinalValue=Holding final value
  spec_Air_tIntkVUs : FromWorkspace  VariableName=testSig_Air_tIntkVUs  Interpolate=off  OutputAfterFinalValue=Holding final value
  spec_CEngDsT_t : FromWorkspace  VariableName=testSig_CEngDsT_t  Interpolate=off  OutputAfterFinalValue=Holding final value
  spec_EngDa_tEng : FromWorkspace  VariableName=testSig_EngDa_tEng  Interpolate=off  OutputAfterFinalValue=Holding final value
  spec_EnvT_t : FromWorkspace  VariableName=testSig_EnvT_t  Interpolate=off  OutputAfterFinalValue=Holding final value
  spec_HPUn_trqLoss : FromWorkspace  VariableName=testSig_HPUn_trqLoss  Interpolate=off  OutputAfterFinalValue=Holding final value
  spec_InjCrv_tAir : FromWorkspace  VariableName=testSig_InjCrv_tAir  Interpolate=off  OutputAfterFinalValue=Holding final value
  spec_InjCrv_tAirMI1 : FromWorkspace  VariableName=testSig_InjCrv_tAirMI1  Interpolate=off  OutputAfterFinalValue=Holding final value
  spec_InjSys_tAir : FromWorkspace  VariableName=testSig_InjSys_tAir  Interpolate=off  OutputAfterFinalValue=Holding final value
  spec_InjSys_tEng : FromWorkspace  VariableName=testSig_InjSys_tEng  Interpolate=off  OutputAfterFinalValue=Holding final value
  spec_InjSys_trqLim : FromWorkspace  VariableName=testSig_InjSys_trqLim  Interpolate=off  OutputAfterFinalValue=Holding final value
  spec_InjSys_trqLoss : FromWorkspace  VariableName=testSig_InjSys_trqLoss  Interpolate=off  OutputAfterFinalValue=Holding final value
  spec_Oil_tSwmp : FromWorkspace  VariableName=testSig_Oil_tSwmp  Interpolate=off  OutputAfterFinalValue=Holding final value
  spec_Rail_tAir : FromWorkspace  VariableName=testSig_Rail_tAir  Interpolate=off  OutputAfterFinalValue=Holding final value
  spec_Rail_trqLim : FromWorkspace  VariableName=testSig_Rail_trqLim  Interpolate=off  OutputAfterFinalValue=Holding final value
  testSignals : Outport
  wires:
  BC/1 -> testSignals/1
  spec_Rail_trqLim/1 -> BC/1  "testSig_Rail_trqLim"
  spec_HPUn_trqLoss/1 -> BC/2  "testSig_HPUn_trqLoss"
  spec_CEngDsT_t/1 -> BC/3  "testSig_CEngDsT_t"
  spec_Oil_tSwmp/1 -> BC/4  "testSig_Oil_tSwmp"
  spec_EngDa_tEng/1 -> BC/5  "testSig_EngDa_tEng"
  spec_Air_tCACDs_mp/1 -> BC/6  "testSig_Air_tCACDs_mp"
  spec_Air_tAFS_mp/1 -> BC/7  "testSig_Air_tAFS_mp"
  spec_EnvT_t/1 -> BC/8  "testSig_EnvT_t"
  spec_Air_tIntkVUs/1 -> BC/9  "testSig_Air_tIntkVUs"
  spec_InjSys_trqLim/1 -> BC/10  "testSig_InjSys_trqLim"
  spec_InjSys_trqLoss/1 -> BC/11  "testSig_InjSys_trqLoss"
  spec_InjSys_tEng/1 -> BC/12  "testSig_InjSys_tEng"
  spec_InjSys_tAir/1 -> BC/13  "testSig_InjSys_tAir"
  spec_Rail_tAir/1 -> BC/14  "testSig_Rail_tAir"
  spec_InjCrv_tAirMI1/1 -> BC/15  "testSig_InjCrv_tAirMI1"
  spec_InjCrv_tAir/1 -> BC/16  "testSig_InjCrv_tAir"

== system TST_InjSys_Co/simulationInput/testSignals_R004 ==
  BC : BusCreator  Inputs=16
  spec_Air_tAFS_mp : FromWorkspace  VariableName=testSig_Air_tAFS_mp  Interpolate=off  OutputAfterFinalValue=Holding final value
  spec_Air_tCACDs_mp : FromWorkspace  VariableName=testSig_Air_tCACDs_mp  Interpolate=off  OutputAfterFinalValue=Holding final value
  spec_Air_tIntkVUs : FromWorkspace  VariableName=testSig_Air_tIntkVUs  Interpolate=off  OutputAfterFinalValue=Holding final value
  spec_CEngDsT_t : FromWorkspace  VariableName=testSig_CEngDsT_t  Interpolate=off  OutputAfterFinalValue=Holding final value
  spec_EngDa_tEng : FromWorkspace  VariableName=testSig_EngDa_tEng  Interpolate=off  OutputAfterFinalValue=Holding final value
  spec_EnvT_t : FromWorkspace  VariableName=testSig_EnvT_t  Interpolate=off  OutputAfterFinalValue=Holding final value
  spec_HPUn_trqLoss : FromWorkspace  VariableName=testSig_HPUn_trqLoss  Interpolate=off  OutputAfterFinalValue=Holding final value
  spec_InjCrv_tAir : FromWorkspace  VariableName=testSig_InjCrv_tAir  Interpolate=off  OutputAfterFinalValue=Holding final value
  spec_InjCrv_tAirMI1 : FromWorkspace  VariableName=testSig_InjCrv_tAirMI1  Interpolate=off  OutputAfterFinalValue=Holding final value
  spec_InjSys_tAir : FromWorkspace  VariableName=testSig_InjSys_tAir  Interpolate=off  OutputAfterFinalValue=Holding final value
  spec_InjSys_tEng : FromWorkspace  VariableName=testSig_InjSys_tEng  Interpolate=off  OutputAfterFinalValue=Holding final value
  spec_InjSys_trqLim : FromWorkspace  VariableName=testSig_InjSys_trqLim  Interpolate=off  OutputAfterFinalValue=Holding final value
  spec_InjSys_trqLoss : FromWorkspace  VariableName=testSig_InjSys_trqLoss  Interpolate=off  OutputAfterFinalValue=Holding final value
  spec_Oil_tSwmp : FromWorkspace  VariableName=testSig_Oil_tSwmp  Interpolate=off  OutputAfterFinalValue=Holding final value
  spec_Rail_tAir : FromWorkspace  VariableName=testSig_Rail_tAir  Interpolate=off  OutputAfterFinalValue=Holding final value
  spec_Rail_trqLim : FromWorkspace  VariableName=testSig_Rail_trqLim  Interpolate=off  OutputAfterFinalValue=Holding final value
  testSignals : Outport
  wires:
  BC/1 -> testSignals/1
  spec_Rail_trqLim/1 -> BC/1  "testSig_Rail_trqLim"
  spec_HPUn_trqLoss/1 -> BC/2  "testSig_HPUn_trqLoss"
  spec_CEngDsT_t/1 -> BC/3  "testSig_CEngDsT_t"
  spec_Oil_tSwmp/1 -> BC/4  "testSig_Oil_tSwmp"
  spec_EngDa_tEng/1 -> BC/5  "testSig_EngDa_tEng"
  spec_Air_tCACDs_mp/1 -> BC/6  "testSig_Air_tCACDs_mp"
  spec_Air_tAFS_mp/1 -> BC/7  "testSig_Air_tAFS_mp"
  spec_EnvT_t/1 -> BC/8  "testSig_EnvT_t"
  spec_Air_tIntkVUs/1 -> BC/9  "testSig_Air_tIntkVUs"
  spec_InjSys_trqLim/1 -> BC/10  "testSig_InjSys_trqLim"
  spec_InjSys_trqLoss/1 -> BC/11  "testSig_InjSys_trqLoss"
  spec_InjSys_tEng/1 -> BC/12  "testSig_InjSys_tEng"
  spec_InjSys_tAir/1 -> BC/13  "testSig_InjSys_tAir"
  spec_Rail_tAir/1 -> BC/14  "testSig_Rail_tAir"
  spec_InjCrv_tAirMI1/1 -> BC/15  "testSig_InjCrv_tAirMI1"
  spec_InjCrv_tAir/1 -> BC/16  "testSig_InjCrv_tAir"

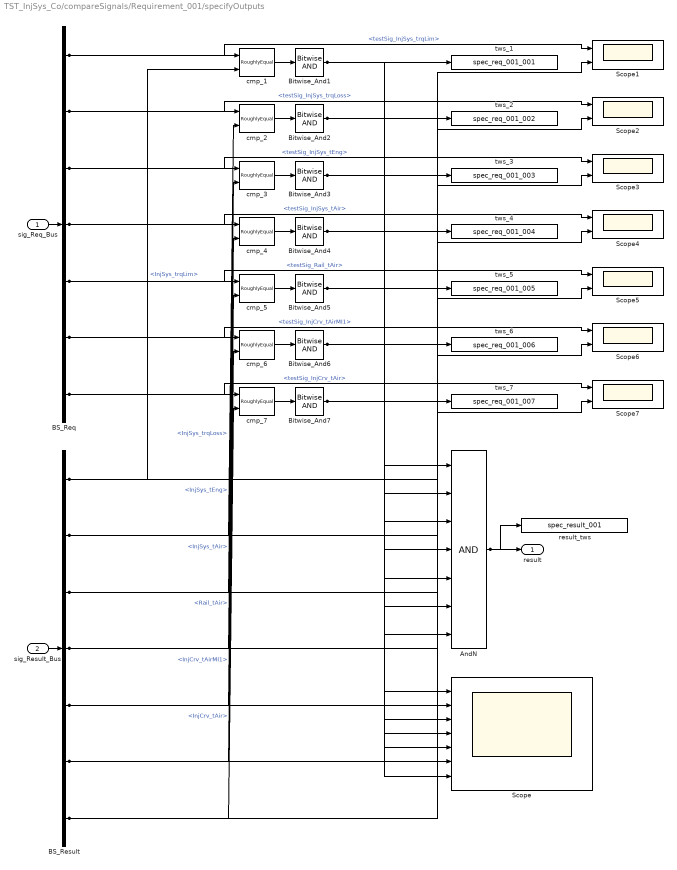
== system TST_InjSys_Co/compareSignals/Requirement_001/specifyOutputs ==
  sig_Req_Bus : Inport
  sig_Result_Bus : Inport  Port=2
  AndN : Logic  Inputs=7
  BS_Req : BusSelector  OutputSignals=testSig_InjSys_trqLim,testSig_InjSys_trqLoss,testSig_InjSys_tEng,testSig_InjSys_tAir,testSig_Rail_tAir,testSig_InjCrv_tAirMI1,testSig_InjCrv_tAir
  BS_Result : BusSelector  OutputSignals=InjSys_trqLim,InjSys_trqLoss,InjSys_tEng,InjSys_tAir,Rail_tAir,InjCrv_tAirMI1,InjCrv_tAir
  Bitwise_And{1..7} (7 alike) : simulink/Logic and Bit Operations/Bitwise Operator  logicop=AND  UseBitMask=off  BitMask=bin2dec('11011001')  BitMaskRealWorld=Stored Integer
  Scope : Scope  NumInputPorts=7
  Scope{1..7} (7 alike) : Scope  NumInputPorts=2
  cmp_{1..7} (7 alike) : UnitTest_Lib/RoughlyEqual  slope=0.1
  result_tws : ToWorkspace  VariableName=spec_result_001
  tws_1 : ToWorkspace  VariableName=spec_req_001_001
  tws_2 : ToWorkspace  VariableName=spec_req_001_002
  tws_3 : ToWorkspace  VariableName=spec_req_001_003
  tws_4 : ToWorkspace  VariableName=spec_req_001_004
  tws_5 : ToWorkspace  VariableName=spec_req_001_005
  tws_6 : ToWorkspace  VariableName=spec_req_001_006
  tws_7 : ToWorkspace  VariableName=spec_req_001_007
  result : Outport
  wires:
  sig_Req_Bus/1 -> BS_Req/1
  sig_Result_Bus/1 -> BS_Result/1
  AndN/1 -> result/1, result_tws/1
  BS_Req/1 -> cmp_1/1, Scope1/1  "<testSig_InjSys_trqLim>"
  BS_Result/1 -> cmp_1/2, Scope1/2  "<InjSys_trqLim>"
  cmp_1/1 -> Bitwise_And1/1
  Bitwise_And1/1 -> tws_1/1, AndN/1, Scope/1
  BS_Req/2 -> cmp_2/1, Scope2/1  "<testSig_InjSys_trqLoss>"
  BS_Result/2 -> cmp_2/2, Scope2/2  "<InjSys_trqLoss>"
  cmp_2/1 -> Bitwise_And2/1
  Bitwise_And2/1 -> tws_2/1, AndN/2, Scope/2
  BS_Req/3 -> cmp_3/1, Scope3/1  "<testSig_InjSys_tEng>"
  BS_Result/3 -> cmp_3/2, Scope3/2  "<InjSys_tEng>"
  cmp_3/1 -> Bitwise_And3/1
  Bitwise_And3/1 -> tws_3/1, AndN/3, Scope/3
  BS_Req/4 -> cmp_4/1, Scope4/1  "<testSig_InjSys_tAir>"
  BS_Result/4 -> cmp_4/2, Scope4/2  "<InjSys_tAir>"
  cmp_4/1 -> Bitwise_And4/1
  Bitwise_And4/1 -> tws_4/1, AndN/4, Scope/4
  BS_Req/5 -> cmp_5/1, Scope5/1  "<testSig_Rail_tAir>"
  BS_Result/5 -> cmp_5/2, Scope5/2  "<Rail_tAir>"
  cmp_5/1 -> Bitwise_And5/1
  Bitwise_And5/1 -> tws_5/1, AndN/5, Scope/5
  BS_Req/6 -> cmp_6/1, Scope6/1  "<testSig_InjCrv_tAirMI1>"
  BS_Result/6 -> cmp_6/2, Scope6/2  "<InjCrv_tAirMI1>"
  cmp_6/1 -> Bitwise_And6/1
  Bitwise_And6/1 -> tws_6/1, AndN/6, Scope/6
  BS_Req/7 -> cmp_7/1, Scope7/1  "<testSig_InjCrv_tAir>"
  BS_Result/7 -> cmp_7/2, Scope7/2  "<InjCrv_tAir>"
  cmp_7/1 -> Bitwise_And7/1
  Bitwise_And7/1 -> tws_7/1, AndN/7, Scope/7

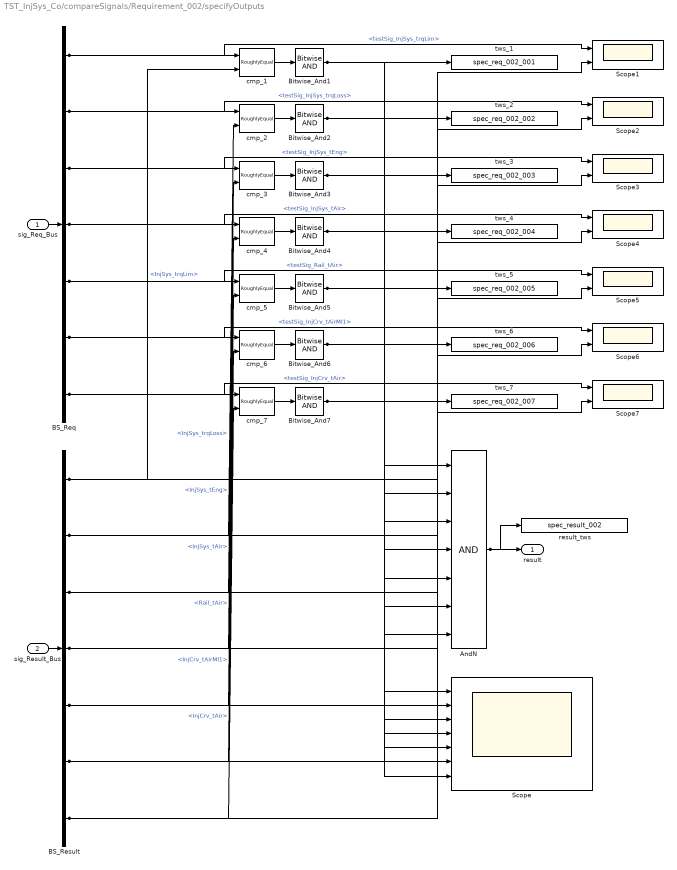
== system TST_InjSys_Co/compareSignals/Requirement_002/specifyOutputs ==
  sig_Req_Bus : Inport
  sig_Result_Bus : Inport  Port=2
  AndN : Logic  Inputs=7
  BS_Req : BusSelector  OutputSignals=testSig_InjSys_trqLim,testSig_InjSys_trqLoss,testSig_InjSys_tEng,testSig_InjSys_tAir,testSig_Rail_tAir,testSig_InjCrv_tAirMI1,testSig_InjCrv_tAir
  BS_Result : BusSelector  OutputSignals=InjSys_trqLim,InjSys_trqLoss,InjSys_tEng,InjSys_tAir,Rail_tAir,InjCrv_tAirMI1,InjCrv_tAir
  Bitwise_And{1..7} (7 alike) : simulink/Logic and Bit Operations/Bitwise Operator  logicop=AND  UseBitMask=off  BitMask=bin2dec('11011001')  BitMaskRealWorld=Stored Integer
  Scope : Scope  NumInputPorts=7
  Scope{1..7} (7 alike) : Scope  NumInputPorts=2
  cmp_{1..7} (7 alike) : UnitTest_Lib/RoughlyEqual  slope=0.1
  result_tws : ToWorkspace  VariableName=spec_result_002
  tws_1 : ToWorkspace  VariableName=spec_req_002_001
  tws_2 : ToWorkspace  VariableName=spec_req_002_002
  tws_3 : ToWorkspace  VariableName=spec_req_002_003
  tws_4 : ToWorkspace  VariableName=spec_req_002_004
  tws_5 : ToWorkspace  VariableName=spec_req_002_005
  tws_6 : ToWorkspace  VariableName=spec_req_002_006
  tws_7 : ToWorkspace  VariableName=spec_req_002_007
  result : Outport
  wires:
  sig_Req_Bus/1 -> BS_Req/1
  sig_Result_Bus/1 -> BS_Result/1
  AndN/1 -> result/1, result_tws/1
  BS_Req/1 -> cmp_1/1, Scope1/1  "<testSig_InjSys_trqLim>"
  BS_Result/1 -> cmp_1/2, Scope1/2  "<InjSys_trqLim>"
  cmp_1/1 -> Bitwise_And1/1
  Bitwise_And1/1 -> tws_1/1, AndN/1, Scope/1
  BS_Req/2 -> cmp_2/1, Scope2/1  "<testSig_InjSys_trqLoss>"
  BS_Result/2 -> cmp_2/2, Scope2/2  "<InjSys_trqLoss>"
  cmp_2/1 -> Bitwise_And2/1
  Bitwise_And2/1 -> tws_2/1, AndN/2, Scope/2
  BS_Req/3 -> cmp_3/1, Scope3/1  "<testSig_InjSys_tEng>"
  BS_Result/3 -> cmp_3/2, Scope3/2  "<InjSys_tEng>"
  cmp_3/1 -> Bitwise_And3/1
  Bitwise_And3/1 -> tws_3/1, AndN/3, Scope/3
  BS_Req/4 -> cmp_4/1, Scope4/1  "<testSig_InjSys_tAir>"
  BS_Result/4 -> cmp_4/2, Scope4/2  "<InjSys_tAir>"
  cmp_4/1 -> Bitwise_And4/1
  Bitwise_And4/1 -> tws_4/1, AndN/4, Scope/4
  BS_Req/5 -> cmp_5/1, Scope5/1  "<testSig_Rail_tAir>"
  BS_Result/5 -> cmp_5/2, Scope5/2  "<Rail_tAir>"
  cmp_5/1 -> Bitwise_And5/1
  Bitwise_And5/1 -> tws_5/1, AndN/5, Scope/5
  BS_Req/6 -> cmp_6/1, Scope6/1  "<testSig_InjCrv_tAirMI1>"
  BS_Result/6 -> cmp_6/2, Scope6/2  "<InjCrv_tAirMI1>"
  cmp_6/1 -> Bitwise_And6/1
  Bitwise_And6/1 -> tws_6/1, AndN/6, Scope/6
  BS_Req/7 -> cmp_7/1, Scope7/1  "<testSig_InjCrv_tAir>"
  BS_Result/7 -> cmp_7/2, Scope7/2  "<InjCrv_tAir>"
  cmp_7/1 -> Bitwise_And7/1
  Bitwise_And7/1 -> tws_7/1, AndN/7, Scope/7

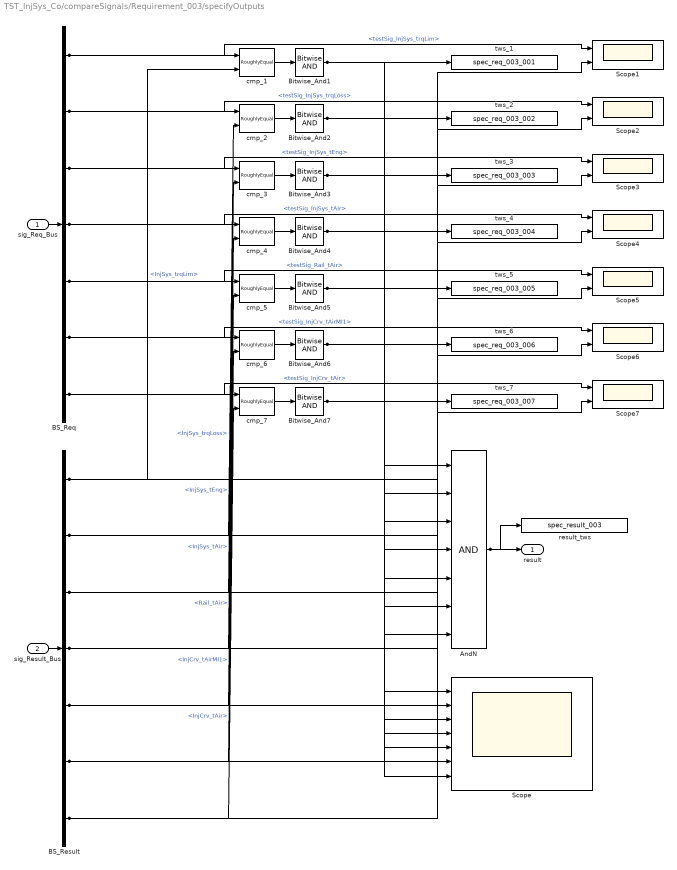
== system TST_InjSys_Co/compareSignals/Requirement_003/specifyOutputs ==
  sig_Req_Bus : Inport
  sig_Result_Bus : Inport  Port=2
  AndN : Logic  Inputs=7
  BS_Req : BusSelector  OutputSignals=testSig_InjSys_trqLim,testSig_InjSys_trqLoss,testSig_InjSys_tEng,testSig_InjSys_tAir,testSig_Rail_tAir,testSig_InjCrv_tAirMI1,testSig_InjCrv_tAir
  BS_Result : BusSelector  OutputSignals=InjSys_trqLim,InjSys_trqLoss,InjSys_tEng,InjSys_tAir,Rail_tAir,InjCrv_tAirMI1,InjCrv_tAir
  Bitwise_And{1..7} (7 alike) : simulink/Logic and Bit Operations/Bitwise Operator  logicop=AND  UseBitMask=off  BitMask=bin2dec('11011001')  BitMaskRealWorld=Stored Integer
  Scope : Scope  NumInputPorts=7
  Scope{1..7} (7 alike) : Scope  NumInputPorts=2
  cmp_{1..7} (7 alike) : UnitTest_Lib/RoughlyEqual  slope=0.1
  result_tws : ToWorkspace  VariableName=spec_result_003
  tws_1 : ToWorkspace  VariableName=spec_req_003_001
  tws_2 : ToWorkspace  VariableName=spec_req_003_002
  tws_3 : ToWorkspace  VariableName=spec_req_003_003
  tws_4 : ToWorkspace  VariableName=spec_req_003_004
  tws_5 : ToWorkspace  VariableName=spec_req_003_005
  tws_6 : ToWorkspace  VariableName=spec_req_003_006
  tws_7 : ToWorkspace  VariableName=spec_req_003_007
  result : Outport
  wires:
  sig_Req_Bus/1 -> BS_Req/1
  sig_Result_Bus/1 -> BS_Result/1
  AndN/1 -> result/1, result_tws/1
  BS_Req/1 -> cmp_1/1, Scope1/1  "<testSig_InjSys_trqLim>"
  BS_Result/1 -> cmp_1/2, Scope1/2  "<InjSys_trqLim>"
  cmp_1/1 -> Bitwise_And1/1
  Bitwise_And1/1 -> tws_1/1, AndN/1, Scope/1
  BS_Req/2 -> cmp_2/1, Scope2/1  "<testSig_InjSys_trqLoss>"
  BS_Result/2 -> cmp_2/2, Scope2/2  "<InjSys_trqLoss>"
  cmp_2/1 -> Bitwise_And2/1
  Bitwise_And2/1 -> tws_2/1, AndN/2, Scope/2
  BS_Req/3 -> cmp_3/1, Scope3/1  "<testSig_InjSys_tEng>"
  BS_Result/3 -> cmp_3/2, Scope3/2  "<InjSys_tEng>"
  cmp_3/1 -> Bitwise_And3/1
  Bitwise_And3/1 -> tws_3/1, AndN/3, Scope/3
  BS_Req/4 -> cmp_4/1, Scope4/1  "<testSig_InjSys_tAir>"
  BS_Result/4 -> cmp_4/2, Scope4/2  "<InjSys_tAir>"
  cmp_4/1 -> Bitwise_And4/1
  Bitwise_And4/1 -> tws_4/1, AndN/4, Scope/4
  BS_Req/5 -> cmp_5/1, Scope5/1  "<testSig_Rail_tAir>"
  BS_Result/5 -> cmp_5/2, Scope5/2  "<Rail_tAir>"
  cmp_5/1 -> Bitwise_And5/1
  Bitwise_And5/1 -> tws_5/1, AndN/5, Scope/5
  BS_Req/6 -> cmp_6/1, Scope6/1  "<testSig_InjCrv_tAirMI1>"
  BS_Result/6 -> cmp_6/2, Scope6/2  "<InjCrv_tAirMI1>"
  cmp_6/1 -> Bitwise_And6/1
  Bitwise_And6/1 -> tws_6/1, AndN/6, Scope/6
  BS_Req/7 -> cmp_7/1, Scope7/1  "<testSig_InjCrv_tAir>"
  BS_Result/7 -> cmp_7/2, Scope7/2  "<InjCrv_tAir>"
  cmp_7/1 -> Bitwise_And7/1
  Bitwise_And7/1 -> tws_7/1, AndN/7, Scope/7

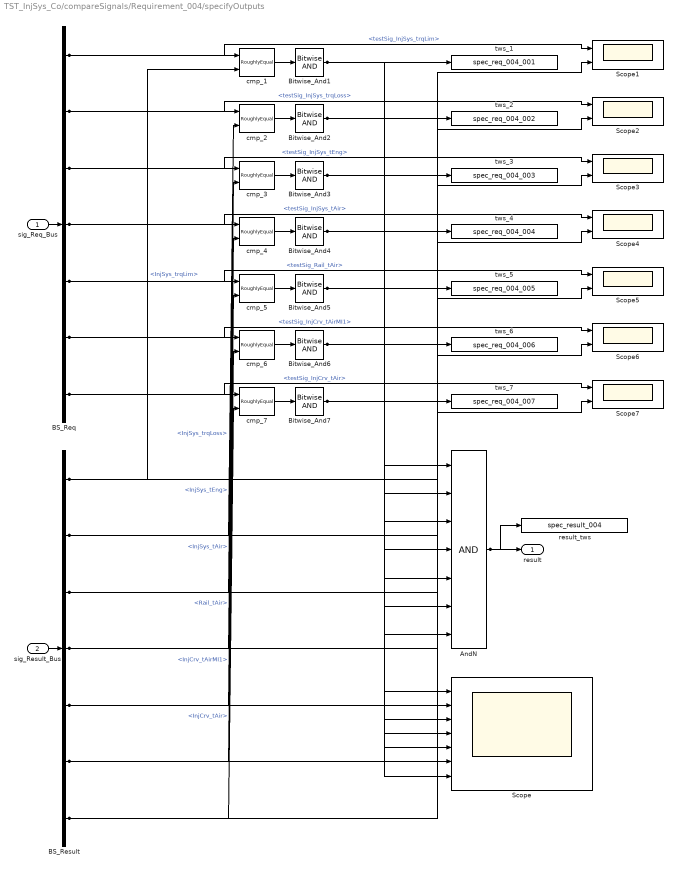
== system TST_InjSys_Co/compareSignals/Requirement_004/specifyOutputs ==
  sig_Req_Bus : Inport
  sig_Result_Bus : Inport  Port=2
  AndN : Logic  Inputs=7
  BS_Req : BusSelector  OutputSignals=testSig_InjSys_trqLim,testSig_InjSys_trqLoss,testSig_InjSys_tEng,testSig_InjSys_tAir,testSig_Rail_tAir,testSig_InjCrv_tAirMI1,testSig_InjCrv_tAir
  BS_Result : BusSelector  OutputSignals=InjSys_trqLim,InjSys_trqLoss,InjSys_tEng,InjSys_tAir,Rail_tAir,InjCrv_tAirMI1,InjCrv_tAir
  Bitwise_And{1..7} (7 alike) : simulink/Logic and Bit Operations/Bitwise Operator  logicop=AND  UseBitMask=off  BitMask=bin2dec('11011001')  BitMaskRealWorld=Stored Integer
  Scope : Scope  NumInputPorts=7
  Scope{1..7} (7 alike) : Scope  NumInputPorts=2
  cmp_{1..7} (7 alike) : UnitTest_Lib/RoughlyEqual  slope=0.1
  result_tws : ToWorkspace  VariableName=spec_result_004
  tws_1 : ToWorkspace  VariableName=spec_req_004_001
  tws_2 : ToWorkspace  VariableName=spec_req_004_002
  tws_3 : ToWorkspace  VariableName=spec_req_004_003
  tws_4 : ToWorkspace  VariableName=spec_req_004_004
  tws_5 : ToWorkspace  VariableName=spec_req_004_005
  tws_6 : ToWorkspace  VariableName=spec_req_004_006
  tws_7 : ToWorkspace  VariableName=spec_req_004_007
  result : Outport
  wires:
  sig_Req_Bus/1 -> BS_Req/1
  sig_Result_Bus/1 -> BS_Result/1
  AndN/1 -> result/1, result_tws/1
  BS_Req/1 -> cmp_1/1, Scope1/1  "<testSig_InjSys_trqLim>"
  BS_Result/1 -> cmp_1/2, Scope1/2  "<InjSys_trqLim>"
  cmp_1/1 -> Bitwise_And1/1
  Bitwise_And1/1 -> tws_1/1, AndN/1, Scope/1
  BS_Req/2 -> cmp_2/1, Scope2/1  "<testSig_InjSys_trqLoss>"
  BS_Result/2 -> cmp_2/2, Scope2/2  "<InjSys_trqLoss>"
  cmp_2/1 -> Bitwise_And2/1
  Bitwise_And2/1 -> tws_2/1, AndN/2, Scope/2
  BS_Req/3 -> cmp_3/1, Scope3/1  "<testSig_InjSys_tEng>"
  BS_Result/3 -> cmp_3/2, Scope3/2  "<InjSys_tEng>"
  cmp_3/1 -> Bitwise_And3/1
  Bitwise_And3/1 -> tws_3/1, AndN/3, Scope/3
  BS_Req/4 -> cmp_4/1, Scope4/1  "<testSig_InjSys_tAir>"
  BS_Result/4 -> cmp_4/2, Scope4/2  "<InjSys_tAir>"
  cmp_4/1 -> Bitwise_And4/1
  Bitwise_And4/1 -> tws_4/1, AndN/4, Scope/4
  BS_Req/5 -> cmp_5/1, Scope5/1  "<testSig_Rail_tAir>"
  BS_Result/5 -> cmp_5/2, Scope5/2  "<Rail_tAir>"
  cmp_5/1 -> Bitwise_And5/1
  Bitwise_And5/1 -> tws_5/1, AndN/5, Scope/5
  BS_Req/6 -> cmp_6/1, Scope6/1  "<testSig_InjCrv_tAirMI1>"
  BS_Result/6 -> cmp_6/2, Scope6/2  "<InjCrv_tAirMI1>"
  cmp_6/1 -> Bitwise_And6/1
  Bitwise_And6/1 -> tws_6/1, AndN/6, Scope/6
  BS_Req/7 -> cmp_7/1, Scope7/1  "<testSig_InjCrv_tAir>"
  BS_Result/7 -> cmp_7/2, Scope7/2  "<InjCrv_tAir>"
  cmp_7/1 -> Bitwise_And7/1
  Bitwise_And7/1 -> tws_7/1, AndN/7, Scope/7
